simulink model "CH06_4"  (R2019a)
settings: Solver=VariableStepAuto  StartTime=0.0  StopTime=10.0  RelTol=1e-3
libraries: simulink x1
settings Model: Creator=吳俊逸  LastModifiedBy=吳俊逸

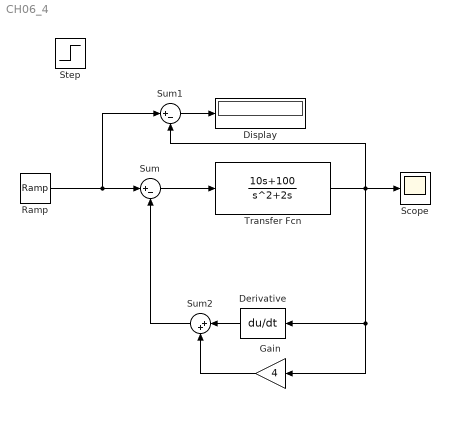
== system CH06_4 ==
  Derivative : Derivative
  Display : Display
  Gain : Gain  Gain=4
  Ramp : simulink/Sources/Ramp  slope=5  start=0  InitialOutput=0
  Scope : Scope
  Step : Step  Time=0  After=5  SampleTime=0
  Sum : Sum  Inputs=|+-
  Sum1 : Sum  Inputs=|+-
  Sum2 : Sum  Inputs=|++
  Transfer Fcn : TransferFcn  Numerator=[10 100]  Denominator=[1 2 0]
  wires:
  Sum/1 -> Transfer Fcn/1
  Transfer Fcn/1 -> Sum1/2, Gain/1, Derivative/1, Scope/1
  Derivative/1 -> Sum2/1
  Gain/1 -> Sum2/2
  Sum2/1 -> Sum/2
  Sum1/1 -> Display/1
  Ramp/1 -> Sum1/1, Sum/1
